simulink model "g_allinone"  (R2021a)
settings: Solver=VariableStepAuto  StartTime=0.0  StopTime=10.0  RelTol=1e-3
settings Model: Creator=Ajay M  LastModifiedBy=Ajay M

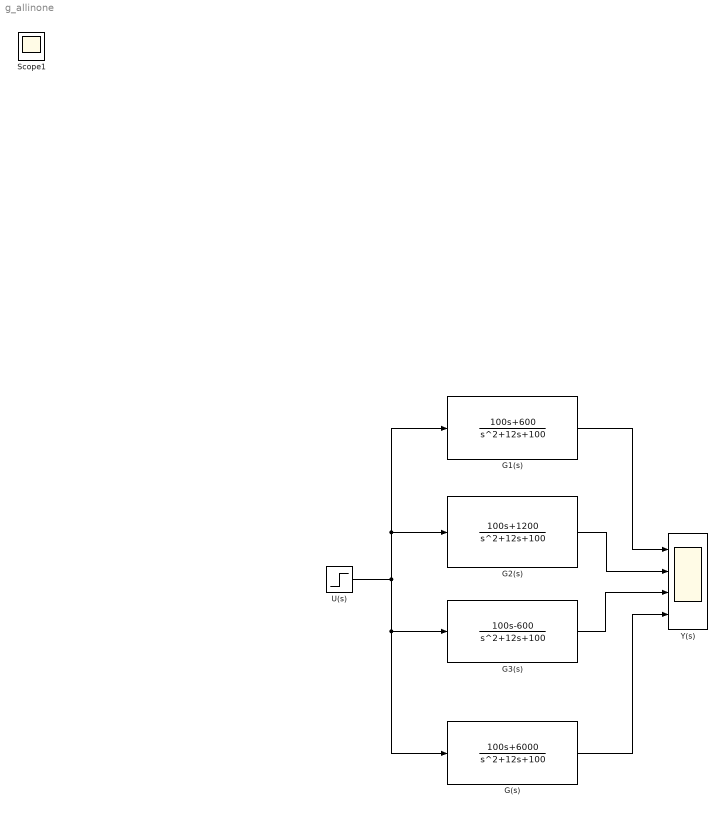
== system g_allinone ==
  G(s) : TransferFcn  Numerator=[100 6000]  Denominator=[1 12 100]
  G1(s) : TransferFcn  Numerator=[100 600]  Denominator=[1 12 100]
  G2(s) : TransferFcn  Numerator=[100 1200]  Denominator=[1 12 100]
  G3(s) : TransferFcn  Numerator=[100 -600]  Denominator=[1 12 100]
  U(s) : Step  SampleTime=0
  Y(s) : Scope  NumInputPorts=4
  Scope1 : Scope
  wires:
  G1(s)/1 -> Y(s)/1
  G2(s)/1 -> Y(s)/2
  G3(s)/1 -> Y(s)/3
  G(s)/1 -> Y(s)/4
  U(s)/1 -> G1(s)/1, G2(s)/1, G3(s)/1, G(s)/1
